simulink model "test2"  (R2022b)
settings: Solver=VariableStepAuto  StartTime=0.0  StopTime=10  RelTol=1e-3
values from neighbouring files (symbols this model uses):
  m_pw = zeros(nvw,nwr)    [fun_getwindpowercurve_v4.m]
  v_beta = 0:1:2    [WGmodel_startup.m]    (also in fun_getwindpowercurve_v2.m = 0.5)
  v_vw = 5:10    [LUT_2D.m]    (also in WGmodel_startup.m = 5:1:10; WGmodel_startup_v2.m = 5:1:15; WGmodel_startup_v3.m = 5:.5:12; fun_getwindpowercurve_v2.m = [10 11 12])
  v_wr = v_Wr/Wrn    [fun_getwindpowercurve.m]    (also in fun_getwindpowercurve_v2.m; fun_getwindpowercurve_v3.m; fun_getwindpowercurve_v4.m; fun_getwindpowercurve_v5.m)
settings Model: Creator=User  LastModifiedBy=User

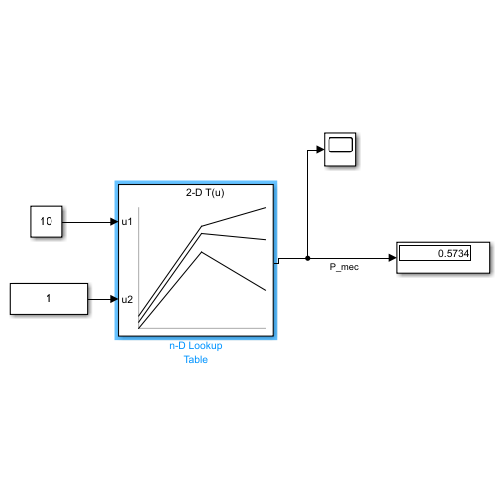
[thumbnail: Simulink's stored preview of the top-level diagram]
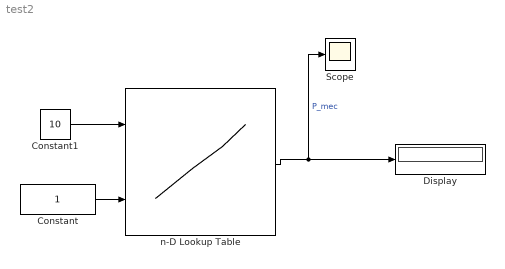
== system test2 ==
  Constant : Constant
  Constant1 : Constant  Value=10
  Display : Display
  Scope : Scope
  n-D Lookup Table : Lookup_n-D  BreakpointsForDimension1=v_vw  BreakpointsForDimension2=v_wr  BreakpointsForDimension3=v_beta  Table=m_pw  InternalRulePriority=Speed  RndMeth=Simplest
      settings: InputPortMap=u0,u1
  wires:
  Constant1/1 -> n-D Lookup Table/1
  Constant/1 -> n-D Lookup Table/2
  n-D Lookup Table/1 -> Scope/1, Display/1  "P_mec"
